simulink model "crs_controller"  (R2025b)
settings: Solver=FixedStepDiscrete  StartTime=0  StopTime=10  FixedStep=0.01  RelTol=1e-3
values from neighbouring files (symbols this model uses):
  brake_threshold = 5.0    [crs_controller.sldd]    (also in crs_controller_params.m = Simulink.Parameter(5);  brake_threshold.DataType = 'single')
  Drv_Override_Hi = 15.0    [crs_controller.sldd]
  Drv_Override_Lo = 5.0    [crs_controller.sldd]
  Kd = -0.0249    [crs_controller.sldd]    (also in crs_controller_params.m = Simulink.Parameter(-0.0249);  Kd.DataType = 'single')
  Ki = 0.2    [crs_controller.sldd]    (also in crs_controller_params.m = Simulink.Parameter(0.2);      Ki.DataType = 'single')
  Kp = 20.0    [crs_controller.sldd]    (also in crs_controller_params.m = Simulink.Parameter(20);       Kp.DataType = 'single')
  press_hold_threshold_samples = 50.0    [crs_controller.sldd]    (also in crs_controller_params.m = Simulink.Parameter(50))
  Spd_Inc_Coarse = 5.0    [crs_controller.sldd]
  Spd_Inc_Fine = 1.0    [crs_controller.sldd]
  Spd_Max = 100.0    [crs_controller.sldd]
  Spd_Min = 40.0    [crs_controller.sldd]
  throttle_max = 100.0    [crs_controller.sldd]    (also in crs_controller_params.m = Simulink.Parameter(100);  throttle_max.DataType = 'single')
  throttle_min = 0.0    [crs_controller.sldd]    (also in crs_controller_params.m = Simulink.Parameter(0);    throttle_min.DataType = 'single')
undefined symbols (not defined in the file or in its folder): opMode
libraries: hdlsllib x14, slpidlib x1
Description:
  | Input: vehicle_speed, driver_throttle, key, enable, cancel, resume, speed_set, inc, dec, brake, gear_drive\nDescription: Cruise Control supervisor and throttle controller\nOutput: throttle_cmd, op_mode, indicator, accel_override, enable_pid
settings Model: DataDictionary=crs_controller.sldd  DNECToolVersion=1.11.0  MATLABVersion=25.2.0.3123386 (R2025b) Update 3  Creator=yasum  LastModifiedBy=yasum
settings DataIOCC: SaveTime=off
settings OptimizationCC: UseDivisionForNetSlopeComputation=on  DefaultUnderspecifiedDataType=single  UseRowMajorAlgorithm=on
settings DebuggingCC: ConsistencyChecking=error  SignalInfNanChecking=error  SignalRangeChecking=error  AlgebraicLoopMsg=error  ArtificialAlgebraicLoopMsg=none  SaveWithDisabledLinksMsg=error  SaveWithParameterizedLinksMsg=error  BlockPriorityViolationMsg=error  TimeAdjustmentMsg=warning  MaxConsecutiveZCsMsg=none  MaskedZcDiagnostic=none  IgnoredZcDiagnostic=none  SolverPrmCheckMsg=error  InheritedTsInSrcMsg=none  SingleTaskRateTransMsg=error  TasksWithSamePriorityMsg=error  CheckMatrixSingularityMsg=error  IntegerOverflowMsg=error  ParameterUnderflowMsg=error  ParameterTunabilityLossMsg=error  UnderSpecifiedDataTypeMsg=error  UnnecessaryDatatypeConvMsg=warning  VectorMatrixConversionMsg=error  SignalLabelMismatchMsg=error  UnconnectedInputMsg=error  UnconnectedOutputMsg=error  UnconnectedLineMsg=error  SFcnCompatibilityMsg=error  BusObjectLabelMismatch=error  RootOutportRequireBusObject=error  AssertControl=DisableAll  UnknownTsInhSupMsg=error  StateNameClashWarn=warning  PregeneratedLibrarySubsystemCodeDiagnostic=none  StrictBusMsg=ErrorOnBusTreatedAsVector  BusNameAdapt=ErrorWithoutRepair  NonBusSignalsTreatedAsBus=error  SFUnusedDataAndEventsDiag=error  SFInvalidInputDataAccessInChartInitDiag=error  SFTransitionOutsideNaturalParentDiag=error  SFUndirectedBroadcastEventsDiag=error  SFTransitionActionBeforeConditionDiag=error  AllowAutomaticUnitConversions=off  VariantConditionMismatch=error
settings ModelReferenceCC: UpdateModelReferenceTargets=IfOutOfDate  EnableRefExpFcnMdlSchedulingChecks=on  ModelReferencePassRootInputsByReference=off
settings SFSimCC: CompileTimeRecursionLimit=0.0  EnableRuntimeRecursion=off  MATLABDynamicMemAlloc=off

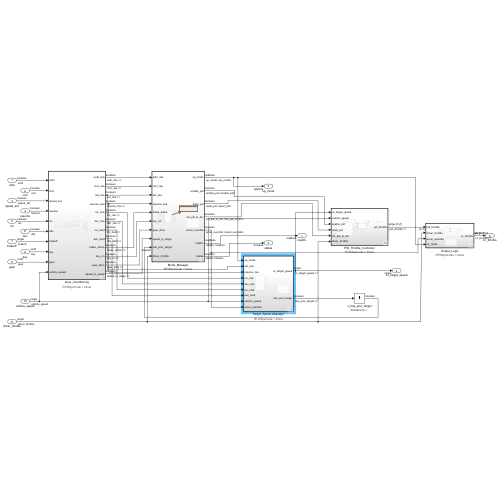
[thumbnail: Simulink's stored preview of the top-level diagram]
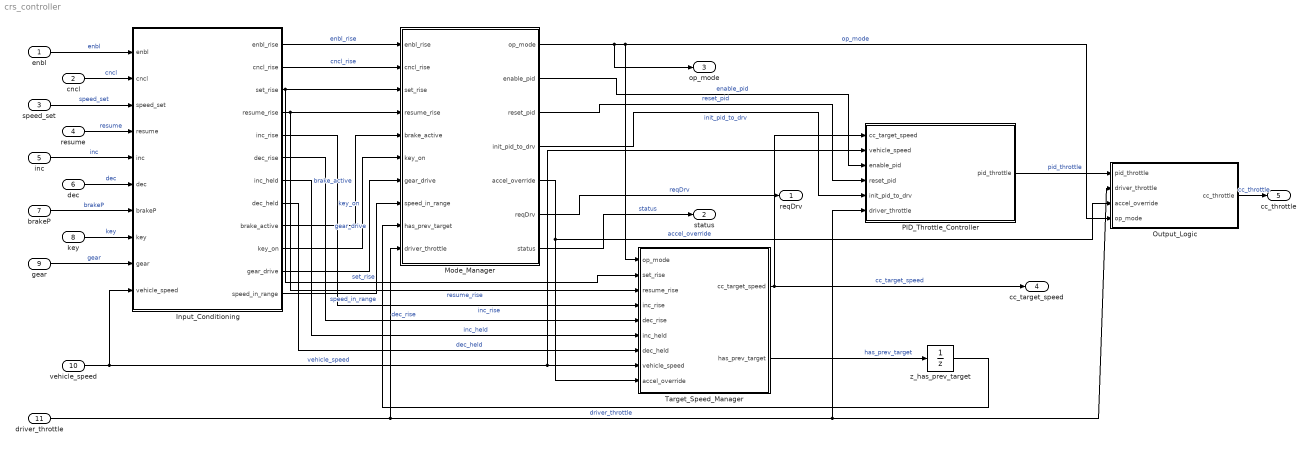
== system crs_controller ==
  enbl : Inport  OutDataTypeStr=boolean
  cncl : Inport  Port=2  OutDataTypeStr=boolean
  speed_set : Inport  Port=3  OutDataTypeStr=boolean
  resume : Inport  Port=4  OutDataTypeStr=boolean
  inc : Inport  Port=5  OutDataTypeStr=boolean
  dec : Inport  Port=6  OutDataTypeStr=boolean
  brakeP : Inport  Port=7  OutDataTypeStr=single
  key : Inport  Port=8  OutDataTypeStr=uint8
  gear : Inport  Port=9  OutDataTypeStr=uint8
  vehicle_speed : Inport  Port=10  OutDataTypeStr=single
  driver_throttle : Inport  Port=11  OutDataTypeStr=single
  Input_Conditioning : Subsystem  Description=Input: vehicle_speed, driver_throttle, enable, cancel, resume, speed_set, inc, dec\nDescription: Edge detection and hold counter processing for driver inputs\nOutput: rise_enable, rise_cncl, rise_resume, speed_set, rise_inc, rise_dec, long_inc, long_dec, vehicle_speed  TreatAsAtomicUnit=on
      settings: AttributesFormatString=RTWSysCode = %<RTWSystemCode>  RTWSystemCode=Inline
  Mode_Manager : Subsystem  Description=Input: rise_enable, rise_cncl, rise_resume, brake, has_prev_target, key, gear_drive\nDescription: Supervisory state machine: Disabled/Enabled/Activated\nOutput: op_mode, reset_pid, init_pid_to_drv, accel_override, enable_pid  TreatAsAtomicUnit=on
      settings: AttributesFormatString=RTWSysCode = %<RTWSystemCode>  RTWSystemCode=Inline
  Output_Logic : Subsystem  Description=Input: op_mode, accel_override, driver_throttle, throttle_cmd\nDescription: Output multiplexing and indicator signal generation\nOutput: throttle_out, indicator, accel_override_out  TreatAsAtomicUnit=on
      settings: AttributesFormatString=RTWSysCode = %<RTWSystemCode>  RTWSystemCode=Inline
  PID_Throttle_Controller : Subsystem  Description=Input: vehicle_speed, cc_target_speed, enable_pid, reset_pid, init_pid_to_drv, driver_throttle\nDescription: Discrete PID throttle controller with anti-windup and bumpless transfer\nOutput: throttle_cmd  TreatAsAtomicUnit=on
      settings: AttributesFormatString=RTWSysCode = %<RTWSystemCode>  RTWSystemCode=Inline
  Target_Speed_Manager : Subsystem  Description=Input: op_mode, vehicle_speed, speed_set, rise_inc, rise_dec, long_inc, long_dec, rise_resume\nDescription: Target cruise speed management with Set/Inc/Dec/Resume logic\nOutput: cc_target_speed, has_prev_target  TreatAsAtomicUnit=on
      settings: AttributesFormatString=RTWSysCode = %<RTWSystemCode>  RTWSystemCode=Inline
  z_has_prev_target : UnitDelay  SampleTime=-1  HasFrameUpgradeWarning=on
      settings: AttributesFormatString=StateName = %<StateName>
  reqDrv : Outport  OutDataTypeStr=Enum: reqMode
  status : Outport  Port=2  OutDataTypeStr=boolean
  op_mode : Outport  Port=3  OutDataTypeStr=Enum: opMode
  cc_target_speed : Outport  Port=4  OutDataTypeStr=single
  cc_throttle : Outport  Port=5  OutDataTypeStr=single
  wires:
  enbl/1 -> Input_Conditioning/1(enbl)  "enbl"
  cncl/1 -> Input_Conditioning/2(cncl)  "cncl"
  Mode_Manager/3(reset_pid) -> PID_Throttle_Controller/4(reset_pid)  "reset_pid"
  gear/1 -> Input_Conditioning/9(gear)  "gear"
  key/1 -> Input_Conditioning/8(key)  "key"
  vehicle_speed/1 -> Target_Speed_Manager/8(vehicle_speed), PID_Throttle_Controller/2(vehicle_speed), Input_Conditioning/10(vehicle_speed)  "vehicle_speed"
  brakeP/1 -> Input_Conditioning/7(brakeP)  "brakeP"
  Mode_Manager/5(accel_override) -> Target_Speed_Manager/9(accel_override), Output_Logic/3(accel_override)  "accel_override"
  speed_set/1 -> Input_Conditioning/3(speed_set)  "speed_set"
  resume/1 -> Input_Conditioning/4(resume)  "resume"
  inc/1 -> Input_Conditioning/5(inc)  "inc"
  dec/1 -> Input_Conditioning/6(dec)  "dec"
  Input_Conditioning/1(enbl_rise) -> Mode_Manager/1(enbl_rise)  "enbl_rise"
  Input_Conditioning/2(cncl_rise) -> Mode_Manager/2(cncl_rise)  "cncl_rise"
  Input_Conditioning/3(set_rise) -> Mode_Manager/3(set_rise), Target_Speed_Manager/2(set_rise)  "set_rise"
  Input_Conditioning/4(resume_rise) -> Mode_Manager/4(resume_rise), Target_Speed_Manager/3(resume_rise)  "resume_rise"
  Input_Conditioning/7(inc_held) -> Target_Speed_Manager/6(inc_held)  "inc_held"
  Input_Conditioning/5(inc_rise) -> Target_Speed_Manager/4(inc_rise)  "inc_rise"
  Input_Conditioning/6(dec_rise) -> Target_Speed_Manager/5(dec_rise)  "dec_rise"
  Input_Conditioning/10(key_on) -> Mode_Manager/6(key_on)  "key_on"
  Input_Conditioning/8(dec_held) -> Target_Speed_Manager/7(dec_held)  "dec_held"
  Target_Speed_Manager/1(cc_target_speed) -> PID_Throttle_Controller/1(cc_target_speed), cc_target_speed/1  "cc_target_speed"
  Input_Conditioning/9(brake_active) -> Mode_Manager/5(brake_active)  "brake_active"
  Input_Conditioning/11(gear_drive) -> Mode_Manager/7(gear_drive)  "gear_drive"
  Input_Conditioning/12(speed_in_range) -> Mode_Manager/8(speed_in_range)  "speed_in_range"
  driver_throttle/1 -> PID_Throttle_Controller/6(driver_throttle), Output_Logic/2(driver_throttle), Mode_Manager/10(driver_throttle)  "driver_throttle"
  Mode_Manager/1(op_mode) -> Target_Speed_Manager/1(op_mode), Output_Logic/4(op_mode), op_mode/1  "op_mode"
  Mode_Manager/2(enable_pid) -> PID_Throttle_Controller/3(enable_pid)  "enable_pid"
  Mode_Manager/6(reqDrv) -> reqDrv/1  "reqDrv"
  Mode_Manager/4(init_pid_to_drv) -> PID_Throttle_Controller/5(init_pid_to_drv)  "init_pid_to_drv"
  Mode_Manager/7(status) -> status/1  "status"
  PID_Throttle_Controller/1(pid_throttle) -> Output_Logic/1(pid_throttle)  "pid_throttle"
  Output_Logic/1(cc_throttle) -> cc_throttle/1  "cc_throttle"
  Target_Speed_Manager/2(has_prev_target) -> z_has_prev_target/1  "has_prev_target"
  z_has_prev_target/1 -> Mode_Manager/9(has_prev_target)

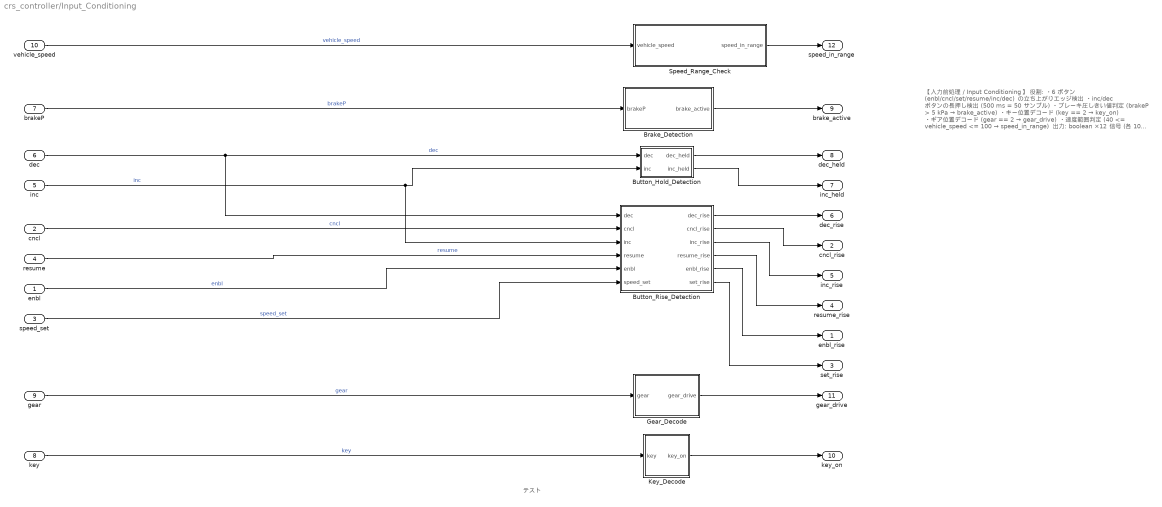
== system crs_controller/Input_Conditioning ==
  note: テスト
  note: 【入力前処理 / Input Conditioning】
      |
      | 役割:
      |   ・6 ボタン (enbl/cncl/set/resume/inc/dec) の立ち上がりエッジ検出
      |   ・inc/dec ボタンの長押し検出 (500 ms = 50 サンプル)
      |   ・ブレーキ圧しきい値判定 (brakeP > 5 kPa → brake_active)
      |   ・キー位置デコード  (key == 2  → key_on)
      |   ・ギア位置デコード  (gear == 2 → gear_drive)
      |   ・速度範囲判定      (40 <= vehicle_speed <= 100 → speed_in_range)
      |
      | 出力: boolean ×12 信号 (各 10 ms サンプル)
  enbl : Inport
  cncl : Inport  Port=2
  speed_set : Inport  Port=3
  resume : Inport  Port=4
  inc : Inport  Port=5
  dec : Inport  Port=6
  brakeP : Inport  Port=7
  key : Inport  Port=8
  gear : Inport  Port=9
  vehicle_speed : Inport  Port=10
  Brake_Detection : Subsystem
  Button_Hold_Detection : Subsystem
  Button_Rise_Detection : Subsystem
  Gear_Decode : Subsystem
  Key_Decode : Subsystem
  Speed_Range_Check : Subsystem
  enbl_rise : Outport
  cncl_rise : Outport  Port=2
  set_rise : Outport  Port=3
  resume_rise : Outport  Port=4
  inc_rise : Outport  Port=5
  dec_rise : Outport  Port=6
  inc_held : Outport  Port=7
  dec_held : Outport  Port=8
  brake_active : Outport  Port=9
  key_on : Outport  Port=10
  gear_drive : Outport  Port=11
  speed_in_range : Outport  Port=12
  wires:
  gear/1 -> Gear_Decode/1(gear)  "gear"
  vehicle_speed/1 -> Speed_Range_Check/1(vehicle_speed)  "vehicle_speed"
  key/1 -> Key_Decode/1(key)  "key"
  brakeP/1 -> Brake_Detection/1(brakeP)  "brakeP"
  dec/1 -> Button_Rise_Detection/1(dec), Button_Hold_Detection/1(dec)  "dec"
  inc/1 -> Button_Hold_Detection/2(inc), Button_Rise_Detection/3(inc)  "inc"
  Brake_Detection/1(brake_active) -> brake_active/1
  cncl/1 -> Button_Rise_Detection/2(cncl)  "cncl"
  resume/1 -> Button_Rise_Detection/4(resume)  "resume"
  enbl/1 -> Button_Rise_Detection/5(enbl)  "enbl"
  speed_set/1 -> Button_Rise_Detection/6(speed_set)  "speed_set"
  Speed_Range_Check/1(speed_in_range) -> speed_in_range/1
  Button_Hold_Detection/1(dec_held) -> dec_held/1
  Button_Hold_Detection/2(inc_held) -> inc_held/1
  Button_Rise_Detection/1(dec_rise) -> dec_rise/1
  Button_Rise_Detection/2(cncl_rise) -> cncl_rise/1
  Button_Rise_Detection/3(inc_rise) -> inc_rise/1
  Button_Rise_Detection/4(resume_rise) -> resume_rise/1
  Button_Rise_Detection/5(enbl_rise) -> enbl_rise/1
  Button_Rise_Detection/6(set_rise) -> set_rise/1
  Gear_Decode/1(gear_drive) -> gear_drive/1
  Key_Decode/1(key_on) -> key_on/1

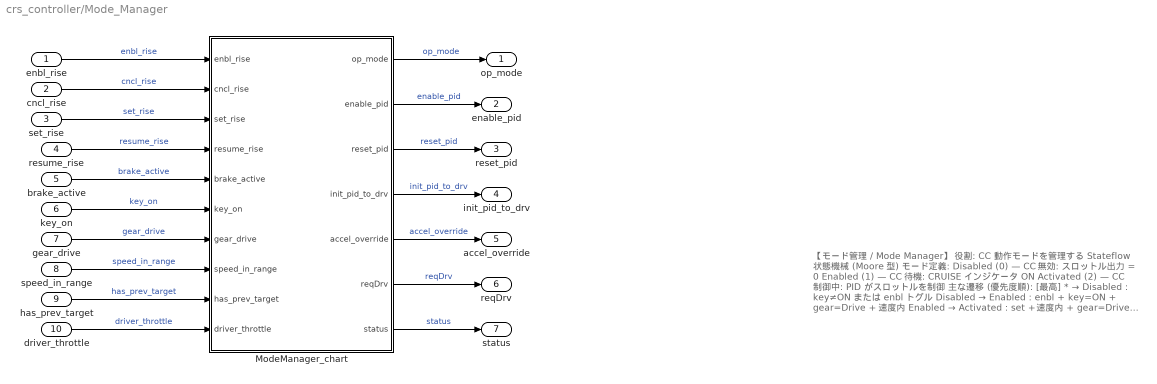
== system crs_controller/Mode_Manager ==
  note: 【モード管理 / Mode Manager】
      |
      | 役割: CC 動作モードを管理する Stateflow 状態機械 (Moore 型)
      |
      | モード定義:
      |   Disabled  (0) — CC 無効: スロットル出力 = 0
      |   Enabled   (1) — CC 待機: CRUISE インジケータ ON
      |   Activated (2) — CC 制御中: PID がスロットルを制御
      |
      | 主な遷移 (優先度順):
      |   [最高] *        → Disabled  : key≠ON または enbl トグル
      |          Disabled → Enabled   : enbl + key=ON + gear=Drive + 速度内
      |          Enabled  → Activated : set + 速度内 + gear=Drive
      |   [低]   Activated→ Enabled   : ブレーキ / cancel / 速度範囲外
      |
      | アクセル操作オーバーライド (Activated 内):
      |   driver_throttle > 15
  enbl_rise : Inport
  cncl_rise : Inport  Port=2
  set_rise : Inport  Port=3
  resume_rise : Inport  Port=4
  brake_active : Inport  Port=5
  key_on : Inport  Port=6
  gear_drive : Inport  Port=7
  speed_in_range : Inport  Port=8
  has_prev_target : Inport  Port=9  OutDataTypeStr=boolean
  driver_throttle : Inport  Port=10
  ModeManager_chart : Stateflow chart  TreatAsAtomicUnit=on
      settings: AttributesFormatString=RTWSysCode = %<RTWSystemCode>
  op_mode : Outport
  enable_pid : Outport  Port=2
  reset_pid : Outport  Port=3
  init_pid_to_drv : Outport  Port=4
  accel_override : Outport  Port=5
  reqDrv : Outport  Port=6
  status : Outport  Port=7
  wires:
  enbl_rise/1 -> ModeManager_chart/1(enbl_rise)  "enbl_rise"
  cncl_rise/1 -> ModeManager_chart/2(cncl_rise)  "cncl_rise"
  key_on/1 -> ModeManager_chart/6(key_on)  "key_on"
  brake_active/1 -> ModeManager_chart/5(brake_active)  "brake_active"
  resume_rise/1 -> ModeManager_chart/4(resume_rise)  "resume_rise"
  set_rise/1 -> ModeManager_chart/3(set_rise)  "set_rise"
  speed_in_range/1 -> ModeManager_chart/8(speed_in_range)  "speed_in_range"
  gear_drive/1 -> ModeManager_chart/7(gear_drive)  "gear_drive"
  has_prev_target/1 -> ModeManager_chart/9(has_prev_target)  "has_prev_target"
  driver_throttle/1 -> ModeManager_chart/10(driver_throttle)  "driver_throttle"
  ModeManager_chart/1(op_mode) -> op_mode/1  "op_mode"
  ModeManager_chart/2(enable_pid) -> enable_pid/1  "enable_pid"
  ModeManager_chart/3(reset_pid) -> reset_pid/1  "reset_pid"
  ModeManager_chart/4(init_pid_to_drv) -> init_pid_to_drv/1  "init_pid_to_drv"
  ModeManager_chart/5(accel_override) -> accel_override/1  "accel_override"
  ModeManager_chart/6(reqDrv) -> reqDrv/1  "reqDrv"
  ModeManager_chart/7(status) -> status/1  "status"

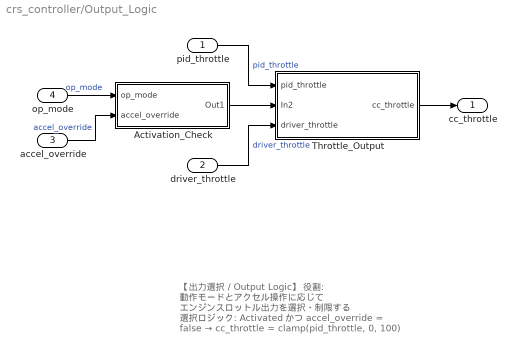
== system crs_controller/Output_Logic ==
  note: 【出力選択 / Output Logic】
      |
      | 役割: 動作モードとアクセル操作に応じて
      |       エンジンスロットル出力を選択・制限する
      |
      | 選択ロジック:
      |   Activated かつ accel_override = false
      |     → cc_throttle = clamp(pid_throttle, 0, 100)
  pid_throttle : Inport
  driver_throttle : Inport  Port=2
  accel_override : Inport  Port=3
  op_mode : Inport  Port=4
  Activation_Check : Subsystem
  Throttle_Output : Subsystem
  cc_throttle : Outport
  wires:
  driver_throttle/1 -> Throttle_Output/3(driver_throttle)  "driver_throttle"
  pid_throttle/1 -> Throttle_Output/1(pid_throttle)  "pid_throttle"
  accel_override/1 -> Activation_Check/2(accel_override)  "accel_override"
  op_mode/1 -> Activation_Check/1(op_mode)  "op_mode"
  Throttle_Output/1(cc_throttle) -> cc_throttle/1
  Activation_Check/1(Out1) -> Throttle_Output/2(In2)

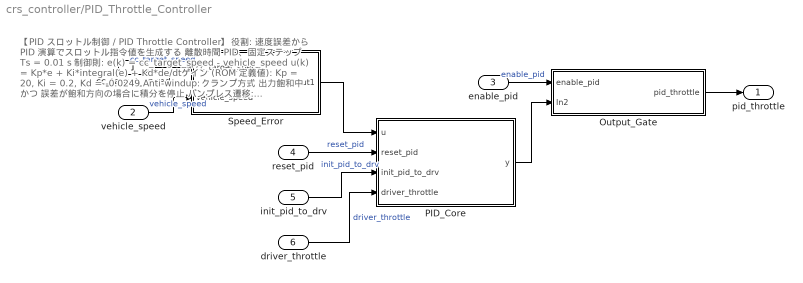
== system crs_controller/PID_Throttle_Controller ==
  note: 【PID スロットル制御 / PID Throttle Controller】
      |
      | 役割: 速度誤差から PID 演算でスロットル指令値を生成する
      |       離散時間 PID、固定ステップ Ts = 0.01 s
      |
      | 制御則:
      |   e(k) = cc_target_speed - vehicle_speed
      |   u(k) = Kp*e + Ki*integral(e) + Kd*de/dt
      |
      | ゲイン (ROM 定義値):
      |   Kp = 20,  Ki = 0.2,  Kd = -0.0249
      |
      | Anti-windup: クランプ方式
      |   出力飽和中 かつ 誤差が飽和方向の場合に積分を停止
      |
      | バンプレス遷移:
      |   Enabled→Activated 移行時: 積分器初期値 = driver_throttle
      |
      | リセット: Disabled 移行時に積分器をクリア
      | 出力範囲: [0, 100]
  cc_target_speed : Inport
  vehicle_speed : Inport  Port=2
  enable_pid : Inport  Port=3
  reset_pid : Inport  Port=4
  init_pid_to_drv : Inport  Port=5
  driver_throttle : Inport  Port=6
  Output_Gate : Subsystem
  PID_Core : Subsystem
  Speed_Error : Subsystem
  pid_throttle : Outport
  wires:
  enable_pid/1 -> Output_Gate/1(enable_pid)  "enable_pid"
  vehicle_speed/1 -> Speed_Error/2(vehicle_speed)  "vehicle_speed"
  driver_throttle/1 -> PID_Core/4(driver_throttle)  "driver_throttle"
  cc_target_speed/1 -> Speed_Error/1(cc_target_speed)  "cc_target_speed"
  init_pid_to_drv/1 -> PID_Core/3(init_pid_to_drv)  "init_pid_to_drv"
  reset_pid/1 -> PID_Core/2(reset_pid)  "reset_pid"
  Speed_Error/1(Out1) -> PID_Core/1(u)
  PID_Core/1(y) -> Output_Gate/2(In2)
  Output_Gate/1(pid_throttle) -> pid_throttle/1

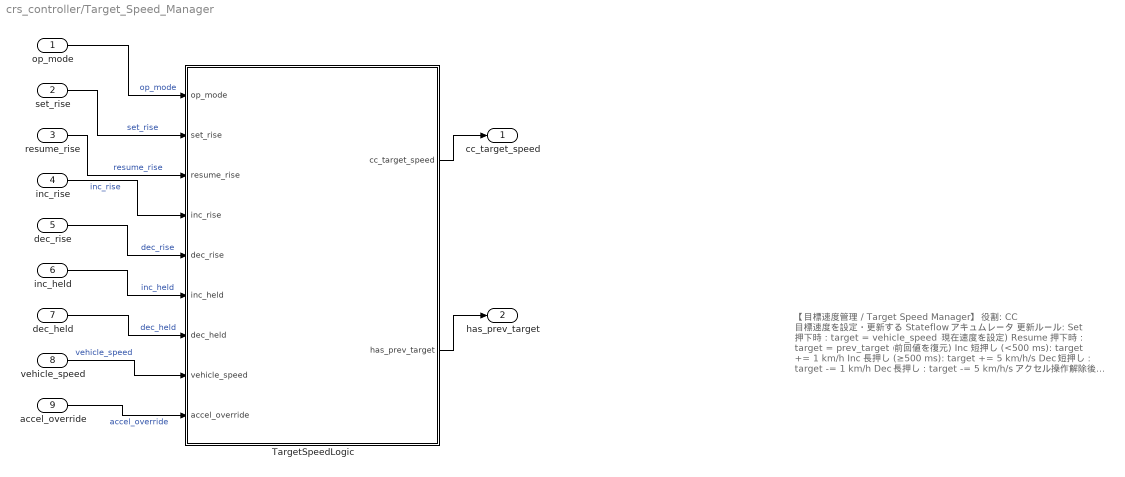
== system crs_controller/Target_Speed_Manager ==
  note: 【目標速度管理 / Target Speed Manager】
      |
      | 役割: CC 目標速度を設定・更新する Stateflow アキュムレータ
      |
      | 更新ルール:
      |   Set 押下時         : target = vehicle_speed (現在速度を設定)
      |   Resume 押下時      : target = prev_target  (前回値を復元)
      |   Inc 短押し (<500 ms): target += 1 km/h
      |   Inc 長押し (≥500 ms): target += 5 km/h/s
      |   Dec 短押し         : target -= 1 km/h
      |   Dec 長押し         : target -= 5 km/h/s
      |   アクセル操作解除後 : target = vehicle_speed (現在速度に更新)
      |
      | 出力範囲: [40, 100] km/h でクランプ
      | 出力: cc_target_speed (single), has_prev_target (boolean)
  op_mode : Inport
  set_rise : Inport  Port=2
  resume_rise : Inport  Port=3
  inc_rise : Inport  Port=4
  dec_rise : Inport  Port=5
  inc_held : Inport  Port=6
  dec_held : Inport  Port=7
  vehicle_speed : Inport  Port=8
  accel_override : Inport  Port=9
  TargetSpeedLogic : Subsystem
  cc_target_speed : Outport
  has_prev_target : Outport  Port=2  OutDataTypeStr=boolean
  wires:
  op_mode/1 -> TargetSpeedLogic/1(op_mode)  "op_mode"
  set_rise/1 -> TargetSpeedLogic/2(set_rise)  "set_rise"
  resume_rise/1 -> TargetSpeedLogic/3(resume_rise)  "resume_rise"
  inc_rise/1 -> TargetSpeedLogic/4(inc_rise)  "inc_rise"
  dec_rise/1 -> TargetSpeedLogic/5(dec_rise)  "dec_rise"
  inc_held/1 -> TargetSpeedLogic/6(inc_held)  "inc_held"
  dec_held/1 -> TargetSpeedLogic/7(dec_held)  "dec_held"
  vehicle_speed/1 -> TargetSpeedLogic/8(vehicle_speed)  "vehicle_speed"
  accel_override/1 -> TargetSpeedLogic/9(accel_override)  "accel_override"
  TargetSpeedLogic/1(cc_target_speed) -> cc_target_speed/1
  TargetSpeedLogic/2(has_prev_target) -> has_prev_target/1

== system crs_controller/Input_Conditioning/Brake_Detection ==
  brakeP : Inport
  ctc_brake : hdlsllib/Logic and Bit Operations/Compare To Constant  relop=>  const=brake_threshold  OutDataTypeStr=boolean
  brake_active : Outport
  wires:
  ctc_brake/1 -> brake_active/1  "brake_active"
  brakeP/1 -> ctc_brake/1

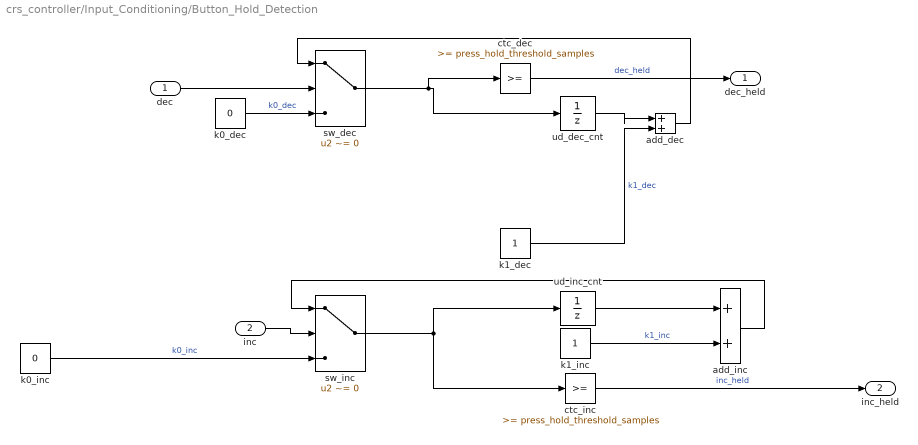
== system crs_controller/Input_Conditioning/Button_Hold_Detection ==
  dec : Inport
  inc : Inport  Port=2
  add_dec : Sum  Inputs=|++  InputSameDT=on  RndMeth=Zero  SaturateOnIntegerOverflow=on
  add_inc : Sum  InputSameDT=on  RndMeth=Zero  SaturateOnIntegerOverflow=on
  ctc_dec : hdlsllib/Logic and Bit Operations/Compare To Constant  relop=>=  const=press_hold_threshold_samples  OutDataTypeStr=boolean
  ctc_inc : hdlsllib/Logic and Bit Operations/Compare To Constant  relop=>=  const=press_hold_threshold_samples  OutDataTypeStr=boolean
  k0_dec : Constant  Value=0  VectorParams1D=off  SampleTime=-1
  k0_inc : Constant  Value=0  VectorParams1D=off  SampleTime=-1
  k1_dec : Constant  VectorParams1D=off  SampleTime=-1
  k1_inc : Constant  VectorParams1D=off  SampleTime=-1
  sw_dec : Switch  Criteria=u2 ~= 0
  sw_inc : Switch  Criteria=u2 ~= 0
  ud_dec_cnt : UnitDelay  SampleTime=-1  HasFrameUpgradeWarning=on
      settings: AttributesFormatString=StateName = %<StateName>
  ud_inc_cnt : UnitDelay  SampleTime=-1  HasFrameUpgradeWarning=on
      settings: AttributesFormatString=StateName = %<StateName>
  dec_held : Outport
  inc_held : Outport  Port=2
  wires:
  ud_inc_cnt/1 -> add_inc/1
  k0_dec/1 -> sw_dec/3  "k0_dec"
  k0_inc/1 -> sw_inc/3  "k0_inc"
  ud_dec_cnt/1 -> add_dec/1
  sw_dec/1 -> ctc_dec/1, ud_dec_cnt/1
  sw_inc/1 -> ctc_inc/1, ud_inc_cnt/1
  k1_inc/1 -> add_inc/2  "k1_inc"
  add_inc/1 -> sw_inc/1
  add_dec/1 -> sw_dec/1
  k1_dec/1 -> add_dec/2  "k1_dec"
  dec/1 -> sw_dec/2
  ctc_dec/1 -> dec_held/1  "dec_held"
  inc/1 -> sw_inc/2
  ctc_inc/1 -> inc_held/1  "inc_held"

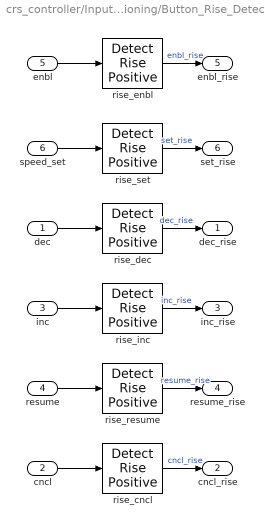
== system crs_controller/Input_Conditioning/Button_Rise_Detection ==
  dec : Inport
  cncl : Inport  Port=2
  inc : Inport  Port=3
  resume : Inport  Port=4
  enbl : Inport  Port=5
  speed_set : Inport  Port=6
  rise_cncl : hdlsllib/Logic and Bit Operations/Detect Rise Positive  vinit=0  OutDataTypeStr=boolean
  rise_dec : hdlsllib/Logic and Bit Operations/Detect Rise Positive  vinit=0  OutDataTypeStr=boolean
  rise_enbl : hdlsllib/Logic and Bit Operations/Detect Rise Positive  vinit=0  OutDataTypeStr=boolean
  rise_inc : hdlsllib/Logic and Bit Operations/Detect Rise Positive  vinit=0  OutDataTypeStr=boolean
  rise_resume : hdlsllib/Logic and Bit Operations/Detect Rise Positive  vinit=0  OutDataTypeStr=boolean
  rise_set : hdlsllib/Logic and Bit Operations/Detect Rise Positive  vinit=0  OutDataTypeStr=boolean
  dec_rise : Outport
  cncl_rise : Outport  Port=2
  inc_rise : Outport  Port=3
  resume_rise : Outport  Port=4
  enbl_rise : Outport  Port=5
  set_rise : Outport  Port=6
  wires:
  enbl/1 -> rise_enbl/1
  dec/1 -> rise_dec/1
  speed_set/1 -> rise_set/1
  inc/1 -> rise_inc/1
  rise_enbl/1 -> enbl_rise/1  "enbl_rise"
  resume/1 -> rise_resume/1
  rise_set/1 -> set_rise/1  "set_rise"
  cncl/1 -> rise_cncl/1
  rise_dec/1 -> dec_rise/1  "dec_rise"
  rise_inc/1 -> inc_rise/1  "inc_rise"
  rise_cncl/1 -> cncl_rise/1  "cncl_rise"
  rise_resume/1 -> resume_rise/1  "resume_rise"

== system crs_controller/Input_Conditioning/Gear_Decode ==
  gear : Inport
  ctc_gear : hdlsllib/Logic and Bit Operations/Compare To Constant  relop===  const=2  OutDataTypeStr=boolean
  gear_drive : Outport
  wires:
  ctc_gear/1 -> gear_drive/1  "gear_drive"
  gear/1 -> ctc_gear/1

== system crs_controller/Input_Conditioning/Key_Decode ==
  key : Inport
  ctc_key : hdlsllib/Logic and Bit Operations/Compare To Constant  relop===  const=2  OutDataTypeStr=boolean
  key_on : Outport
  wires:
  ctc_key/1 -> key_on/1  "key_on"
  key/1 -> ctc_key/1

== system crs_controller/Input_Conditioning/Speed_Range_Check ==
  vehicle_speed : Inport
  and_spd : Logic  IconShape=distinctive  OutDataTypeStr=boolean
  ctc_spd_hi : hdlsllib/Logic and Bit Operations/Compare To Constant  relop=<=  const=Spd_Max  OutDataTypeStr=boolean
  ctc_spd_lo : hdlsllib/Logic and Bit Operations/Compare To Constant  relop=>=  const=Spd_Min  OutDataTypeStr=boolean
  speed_in_range : Outport
  wires:
  vehicle_speed/1 -> ctc_spd_hi/1, ctc_spd_lo/1
  ctc_spd_hi/1 -> and_spd/2
  ctc_spd_lo/1 -> and_spd/1
  and_spd/1 -> speed_in_range/1  "speed_in_range"

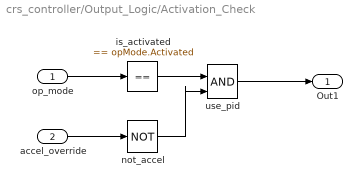
== system crs_controller/Output_Logic/Activation_Check ==
  op_mode : Inport
  accel_override : Inport  Port=2
  is_activated : hdlsllib/Logic and Bit Operations/Compare To Constant  relop===  const=opMode.Activated  OutDataTypeStr=boolean
  not_accel : Logic  Operator=NOT  Inputs=1  IconShape=distinctive  OutDataTypeStr=boolean
  use_pid : Logic  IconShape=distinctive  OutDataTypeStr=boolean
  Out1 : Outport
  wires:
  is_activated/1 -> use_pid/1
  not_accel/1 -> use_pid/2
  op_mode/1 -> is_activated/1
  accel_override/1 -> not_accel/1
  use_pid/1 -> Out1/1

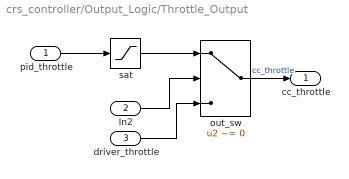
== system crs_controller/Output_Logic/Throttle_Output ==
  pid_throttle : Inport
  In2 : Inport  Port=2
  driver_throttle : Inport  Port=3
  out_sw : Switch  Criteria=u2 ~= 0
  sat : Saturate  UpperLimit=throttle_max  LowerLimit=throttle_min
      settings: AttributesFormatString=|
      | UpperLimit = %<UpperLimit>
      | LowerLimit = %<LowerLimit>
  cc_throttle : Outport
  wires:
  pid_throttle/1 -> sat/1
  out_sw/1 -> cc_throttle/1  "cc_throttle"
  sat/1 -> out_sw/1
  In2/1 -> out_sw/2
  driver_throttle/1 -> out_sw/3

== system crs_controller/PID_Throttle_Controller/Output_Gate ==
  enable_pid : Inport
  In2 : Inport  Port=2
  k_zero : Constant  Value=single(0)  VectorParams1D=off  SampleTime=-1
  sw_enable : Switch  Criteria=u2 ~= 0
  pid_throttle : Outport
  wires:
  k_zero/1 -> sw_enable/3
  In2/1 -> sw_enable/1
  enable_pid/1 -> sw_enable/2
  sw_enable/1 -> pid_throttle/1  "pid_throttle"

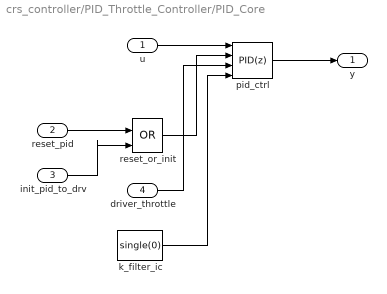
== system crs_controller/PID_Throttle_Controller/PID_Core ==
  u : Inport
  reset_pid : Inport  Port=2
  init_pid_to_drv : Inport  Port=3
  driver_throttle : Inport  Port=4
  k_filter_ic : Constant  Value=single(0)  VectorParams1D=off  SampleTime=-1
  pid_ctrl : slpidlib/PID Controller  Controller=PID  Form=Parallel  TimeDomain=Discrete-time  UseExternalTs=off  SampleTime=-1  IntegratorMethod=Forward Euler  FilterMethod=Forward Euler  ControllerParametersSource=internal  P=Kp  I=Ki  UseKiTs=off  D=Kd  UseExternalDerivativeSource=off  N=100  UseFilter=on  TunerSelectOption=Transfer Function Based (PID Tuner App)  InitialConditionSource=external  InitialConditionForIntegrator=0  InitialConditionForFilter=0  DifferentiatorICPrevScaledInput=0  ExternalReset=rising  TrackingMode=off  Kt=1  LimitOutput=off  SatLimitsSource=internal  UpperSaturationLimit=100  LowerSaturationLimit=0  LinearizeAsGain=off  AntiWindupMode=clamping  Kb=1  LimitIntegrator=off  UpperIntegratorSaturationLimit=inf  LowerIntegratorSaturationLimit=-inf  POutMin=[]  POutMax=[]  IOutMin=[]  IOutMax=[]  DOutMin=[]  DOutMax=[]  NOutMin=[]  NOutMax=[]  SumOutMin=[]  SumOutMax=[]  SaturationOutMin=[]  SaturationOutMax=[]  PParamMin=[]  PParamMax=[]  IParamMin=[]  IParamMax=[]  DParamMin=[]  DParamMax=[]  NParamMin=[]  NParamMax=[]  KbParamMin=[]  KbParamMax=[]  KtParamMin=[]  KtParamMax=[]  KbOutMin=[]  KbOutMax=[]  KtOutMin=[]  KtOutMax=[]  IntegratorOutMin=[]  IntegratorOutMax=[]  FilterOutMin=[]  FilterOutMax=[]  SumI1OutMin=[]  SumI1OutMax=[]  SumI2OutMin=[]  SumI2OutMax=[]  SumI3OutMin=[]  SumI3OutMax=[]  SumI4OutMin=[]  SumI4OutMax=[]  SumDOutMin=[]  SumDOutMax=[]  DifferentiatorOutMin=[]  DifferentiatorOutMax=[]  FilterDiffOutCoefMin=[]  FilterDiffOutCoefMax=[]  ReciprocalOutMin=[]  ReciprocalOutMax=[]  SumDenOutMin=[]  SumDenOutMax=[]  SumNumOutMin=[]  SumNumOutMax=[]  DivideOutMin=[]  DivideOutMax=[]  UdiffTsProdOutMin=[]  UdiffTsProdOutMax=[]  NTsProdOutMin=[]  NTsProdOutMax=[]  UintegralTsProdOutMin=[]  UintegralTsProdOutMax=[]  UngainTsProdOutMin=[]  UngainTsProdOutMax=[]  ClampingZeroOutDataTypeStr=Inherit: Inherit via back propagation  ClampingZeroOutMin=[]  ClampingZeroOutMax=[]  FilterDenConstantOutDataTypeStr=Inherit: Inherit via back propagation  FilterDenConstantOutMin=[]  FilterDenConstantOutMax=[]  PCopyOutDataTypeStr=Inherit: Inherit via back propagation  PCopyOutMin=[]  PCopyOutMax=[]  NCopyOutDataTypeStr=Inherit: Inherit via back propagation  NCopyOutMin=[]  NCopyOutMax=[]  IntegratorContinuousStateAttributes=''  IntegratorStateMustResolveToSignalObject=off  IntegratorRTWStateStorageClass=Auto  FilterContinuousStateAttributes=''  FilterStateMustResolveToSignalObject=off  FilterRTWStateStorageClass=Auto  ParallelPVariant=InternalParameters  IdealPVariant=Disabled  IVariant=InternalParameters  DVariant=InternalParameters  IntegratorVariant=Discrete  SatVariant=Disabled  AWVariant=Passthrough  PCopyVariant=Disabled  TRVariant=Disabled  FdbkBlocksVariant=Forward  IdealPFdbkVariant=Disabled  SatFdbkVariant=Disabled  DerivativeFilterVariant=ForwardEulerFilter  NVariant=InternalParameters  NCopyVariant=Disabled  FilterICVariant=ExternalICs  IntegratorICVariant=ExternalICs  ExternalResetVariant=ExternalReset  TRSumVariant=Passthrough  SumFdbkVariant=Disabled  SumVariant=Sum_PID  TsampFilterVariant=InternalTs  TsampNgainVariant=Passthrough  TsampIntegralVariant=Disabled_SignalSpec  ExternalSaturationOutDataTypeStr=Inherit: Same as second input  DerivativeSourceVariant=ErrorSignal  PreIntVariant=InternalPreInt
      settings: LibrarySourceBlock=hdlsllib/Discrete/Discrete PID Controller
  reset_or_init : Logic  Operator=OR  IconShape=distinctive  OutDataTypeStr=boolean
  y : Outport
  wires:
  reset_or_init/1 -> pid_ctrl/2
  k_filter_ic/1 -> pid_ctrl/4
  reset_pid/1 -> reset_or_init/1
  init_pid_to_drv/1 -> reset_or_init/2
  driver_throttle/1 -> pid_ctrl/3
  pid_ctrl/1 -> y/1
  u/1 -> pid_ctrl/1

== system crs_controller/PID_Throttle_Controller/Speed_Error ==
  cc_target_speed : Inport
  vehicle_speed : Inport  Port=2
  err_sum : Sum  Inputs=+-  InputSameDT=on  RndMeth=Zero  SaturateOnIntegerOverflow=on
  Out1 : Outport
  wires:
  err_sum/1 -> Out1/1
  vehicle_speed/1 -> err_sum/2
  cc_target_speed/1 -> err_sum/1

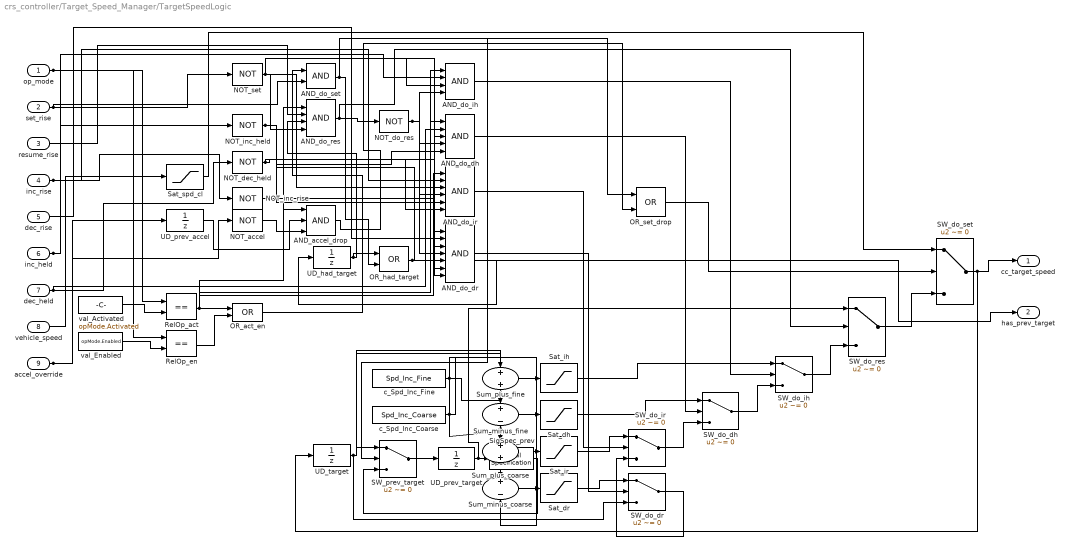
== system crs_controller/Target_Speed_Manager/TargetSpeedLogic ==
  op_mode : Inport
  set_rise : Inport  Port=2
  resume_rise : Inport  Port=3
  inc_rise : Inport  Port=4
  dec_rise : Inport  Port=5
  inc_held : Inport  Port=6
  dec_held : Inport  Port=7
  vehicle_speed : Inport  Port=8
  accel_override : Inport  Port=9
  AND_accel_drop : Logic  Inputs=3  AllPortsSameDT=off  OutDataTypeStr=boolean
  AND_do_dh : Logic  Inputs=5  AllPortsSameDT=off  OutDataTypeStr=boolean
  AND_do_dr : Logic  Inputs=7  AllPortsSameDT=off  OutDataTypeStr=boolean
  AND_do_ih : Logic  Inputs=4  AllPortsSameDT=off  OutDataTypeStr=boolean
  AND_do_ir : Logic  Inputs=6  AllPortsSameDT=off  OutDataTypeStr=boolean
  AND_do_res : Logic  Inputs=4  AllPortsSameDT=off  OutDataTypeStr=boolean
  AND_do_set : Logic  AllPortsSameDT=off  OutDataTypeStr=boolean
  NOT_accel : Logic  Operator=NOT  AllPortsSameDT=off  OutDataTypeStr=boolean
  NOT_dec_held : Logic  Operator=NOT  AllPortsSameDT=off  OutDataTypeStr=boolean
  NOT_do_res : Logic  Operator=NOT  AllPortsSameDT=off  OutDataTypeStr=boolean
  NOT_inc_held : Logic  Operator=NOT  AllPortsSameDT=off  OutDataTypeStr=boolean
  NOT_inc_rise : Logic  Operator=NOT  AllPortsSameDT=off  OutDataTypeStr=boolean
  NOT_set : Logic  Operator=NOT  AllPortsSameDT=off  OutDataTypeStr=boolean
  OR_act_en : Logic  Operator=OR  AllPortsSameDT=off  OutDataTypeStr=boolean
  OR_had_target : Logic  Operator=OR  AllPortsSameDT=off  OutDataTypeStr=boolean
  OR_set_drop : Logic  Operator=OR  AllPortsSameDT=off  OutDataTypeStr=boolean
  RelOp_act : RelationalOperator  Operator===  OutDataTypeStr=boolean  RndMeth=Simplest  InputSameDT=off
  RelOp_en : RelationalOperator  Operator===  OutDataTypeStr=boolean  RndMeth=Simplest  InputSameDT=off
  SW_do_dh : Switch  Criteria=u2 ~= 0  SaturateOnIntegerOverflow=off  InputSameDT=off
  SW_do_dr : Switch  Criteria=u2 ~= 0  SaturateOnIntegerOverflow=off  InputSameDT=off
  SW_do_ih : Switch  Criteria=u2 ~= 0  SaturateOnIntegerOverflow=off  InputSameDT=off
  SW_do_ir : Switch  Criteria=u2 ~= 0  SaturateOnIntegerOverflow=off  InputSameDT=off
  SW_do_res : Switch  Criteria=u2 ~= 0  SaturateOnIntegerOverflow=off  InputSameDT=off
  SW_do_set : Switch  Criteria=u2 ~= 0  SaturateOnIntegerOverflow=off  InputSameDT=off
  SW_prev_target : Switch  Criteria=u2 ~= 0  SaturateOnIntegerOverflow=off  InputSameDT=off
  Sat_dh : Saturate  UpperLimit=Spd_Max  LowerLimit=Spd_Min
  Sat_dr : Saturate  UpperLimit=Spd_Max  LowerLimit=Spd_Min
  Sat_ih : Saturate  UpperLimit=Spd_Max  LowerLimit=Spd_Min
  Sat_ir : Saturate  UpperLimit=Spd_Max  LowerLimit=Spd_Min
  Sat_spd_cl : Saturate  UpperLimit=Spd_Max  LowerLimit=Spd_Min
  SigSpec_prev : SignalSpecification  OutDataTypeStr=single  Dimensions=1
  Sum_minus_coarse : Sum  Inputs=+-
  Sum_minus_fine : Sum  Inputs=+-
  Sum_plus_coarse : Sum
  Sum_plus_fine : Sum
  UD_had_target : UnitDelay  InitialCondition=false  SampleTime=-1  HasFrameUpgradeWarning=on
  UD_prev_accel : UnitDelay  InitialCondition=false  SampleTime=-1  HasFrameUpgradeWarning=on
  UD_prev_target : UnitDelay  InitialCondition=single(0)  SampleTime=-1  HasFrameUpgradeWarning=on
  UD_target : UnitDelay  InitialCondition=single(0)  SampleTime=-1  HasFrameUpgradeWarning=on
  c_Spd_Inc_Coarse : Constant  Value=Spd_Inc_Coarse  OutDataTypeStr=single
  c_Spd_Inc_Fine : Constant  Value=Spd_Inc_Fine  OutDataTypeStr=single
  val_Activated : Constant  Value=opMode.Activated  OutDataTypeStr=Enum: opMode
  val_Enabled : Constant  Value=opMode.Enabled  OutDataTypeStr=Enum: opMode
  cc_target_speed : Outport
  has_prev_target : Outport  Port=2
  wires:
  op_mode/1 -> RelOp_act/1, RelOp_en/1
  val_Activated/1 -> RelOp_act/2
  val_Enabled/1 -> RelOp_en/2
  RelOp_act/1 -> OR_act_en/1, AND_accel_drop/1, AND_do_res/1, AND_do_ih/1, AND_do_dh/1, AND_do_ir/1, AND_do_dr/1
  RelOp_en/1 -> OR_act_en/2
  vehicle_speed/1 -> Sat_spd_cl/1
  accel_override/1 -> UD_prev_accel/1, NOT_accel/1
  UD_prev_accel/1 -> AND_accel_drop/2
  NOT_accel/1 -> AND_accel_drop/3
  set_rise/1 -> NOT_set/1, AND_do_set/2
  inc_held/1 -> NOT_inc_held/1, AND_do_ih/2
  dec_held/1 -> NOT_dec_held/1, AND_do_dh/2
  inc_rise/1 -> NOT_inc_rise/1, AND_do_ir/2
  OR_act_en/1 -> AND_do_set/1
  resume_rise/1 -> AND_do_res/2
  UD_had_target/1 -> AND_do_res/3, OR_had_target/1
  NOT_set/1 -> AND_do_res/4, AND_do_ih/3, AND_do_dh/3, AND_do_ir/3, AND_do_dr/3
  AND_do_res/1 -> NOT_do_res/1, SW_do_res/2
  NOT_do_res/1 -> AND_do_ih/4, AND_do_dh/4, AND_do_ir/4, AND_do_dr/4
  NOT_inc_held/1 -> AND_do_dh/5, AND_do_ir/5, AND_do_dr/5
  NOT_dec_held/1 -> AND_do_ir/6, AND_do_dr/6
  dec_rise/1 -> AND_do_dr/2
  NOT_inc_rise/1 -> AND_do_dr/7
  AND_do_set/1 -> OR_had_target/2, SW_prev_target/2, OR_set_drop/1
  OR_had_target/1 -> UD_had_target/1, has_prev_target/1
  UD_target/1 -> SW_prev_target/1, Sum_plus_fine/1, Sum_minus_fine/1, Sum_plus_coarse/1, Sum_minus_coarse/1, SW_do_dr/3
  UD_prev_target/1 -> SW_do_res/1, SigSpec_prev/1
  SW_prev_target/1 -> UD_prev_target/1
  c_Spd_Inc_Fine/1 -> Sum_plus_fine/2, Sum_minus_fine/2
  c_Spd_Inc_Coarse/1 -> Sum_plus_coarse/2, Sum_minus_coarse/2
  Sum_plus_fine/1 -> Sat_ih/1
  Sum_minus_fine/1 -> Sat_dh/1
  Sum_plus_coarse/1 -> Sat_ir/1
  Sum_minus_coarse/1 -> Sat_dr/1
  Sat_dr/1 -> SW_do_dr/1
  AND_do_dr/1 -> SW_do_dr/2
  Sat_ir/1 -> SW_do_ir/1
  AND_do_ir/1 -> SW_do_ir/2
  SW_do_dr/1 -> SW_do_ir/3
  Sat_dh/1 -> SW_do_dh/1
  AND_do_dh/1 -> SW_do_dh/2
  SW_do_ir/1 -> SW_do_dh/3
  Sat_ih/1 -> SW_do_ih/1
  AND_do_ih/1 -> SW_do_ih/2
  SW_do_dh/1 -> SW_do_ih/3
  SW_do_ih/1 -> SW_do_res/3
  AND_accel_drop/1 -> OR_set_drop/2
  Sat_spd_cl/1 -> SW_do_set/1
  OR_set_drop/1 -> SW_do_set/2
  SW_do_res/1 -> SW_do_set/3
  SW_do_set/1 -> cc_target_speed/1, UD_target/1
  SigSpec_prev/1 -> SW_prev_target/3

== stateflow chart crs_controller/Mode_Manager/ModeManager_chart ==
  settings: updateMethod=DISCRETE  sampleTime=0.01
  state Enabled
    entry:
    op_mode=opMode.Enabled; enable_pid=false; reset_pid=false;
    init_pid_to_drv=false; accel_override=false;
    reqDrv=reqMode.None; status=true; prev_accel_ov=false;
  state Disabled
    entry:
    op_mode=opMode.Disabled; enable_pid=false; reset_pid=true;
    init_pid_to_drv=false; accel_override=false;
    reqDrv=reqMode.None; status=false; prev_accel_ov=false;
  state Activated
    entry:
    op_mode=opMode.Activated; reset_pid=false; init_pid_to_drv=true;
    accel_override=false; prev_accel_ov=false;
    reqDrv=reqMode.None; status=true; enable_pid=true;
    during:
    init_pid_to_drv=false;
    // Accel override hysteresis:
    //   override_start: throttle > Drv_Override_Hi  -> override begins
    //   override_hold : prev override ON AND throttle >= Drv_Override_Lo -> override sustained
    prev_accel_ov = (driver_throttle > Drv_Override_Hi) || (prev_accel_ov && (driver_throttle >= Drv_Override_Lo));
    accel_override = prev_accel_ov;
    enable_pid = !prev_accel_ov;
  (default) -> Disabled
  Disabled -> Enabled : [enbl_rise && key_on && gear_drive]{reqDrv=reqMode.EnableReq;}
  Enabled -> Disabled [order 2] : [!key_on || enbl_rise]{reqDrv=reqMode.DisableReq;}
  Enabled -> Activated [order 1] : [set_rise && speed_in_range && gear_drive]{reqDrv=reqMode.ActivateReq;}
  Enabled -> Activated [order 3] : [resume_rise && has_prev_target && speed_in_range && gear_drive]{reqDrv=reqMode.ResumeReq;}
  Activated -> Enabled [order 2] : [brake_active || cncl_rise || !gear_drive || !speed_in_range]{reqDrv=reqMode.DeactivateReq;}
  Activated -> Disabled [order 1] : [!key_on || enbl_rise]{reqDrv=reqMode.DisableReq;}
  data: enbl_rise input boolean; cncl_rise input boolean; set_rise input boolean; resume_rise input boolean; brake_active input boolean; key_on input boolean; gear_drive input boolean; speed_in_range input boolean; has_prev_target input boolean; driver_throttle input single; op_mode output Enum: opMode size=1; enable_pid output boolean size=1; reset_pid output boolean size=1; init_pid_to_drv output boolean size=1; accel_override output boolean size=1; reqDrv output Enum: reqMode size=1; status output boolean size=1; prev_accel_ov local boolean size=1 =false; Drv_Override_Hi parameter single size=1; Drv_Override_Lo parameter single size=1
